simulink model "SistemaLineal"  (R2018b)
settings: Solver=VariableStepAuto  StartTime=0.0  StopTime=ttotal  RelTol=1e-3
values from neighbouring files (symbols this model uses):
  denom = conv(conv(conv([1 0.2], [1 -0.6]),[1 0.4]),[1 -0.1])    [PruebaMinCuadrados.m]
  num = conv(conv(conv([1 0.5], [1 0.7]),[1 -0.2]),[0 1])    [PruebaMinCuadrados.m]
  tmuestra = 0.05    [IDDATA.m]    (also in Identificacion.m; PruebaMinCuadrados.m)
  var = 0.00001    (= 1e-05)    [Identificacion.m]    (also in PruebaMinCuadrados.m = 0.001)
undefined symbols (not defined in the file or in its folder): iseed
settings Model: Creator=pablo  LastModifiedBy=pablo

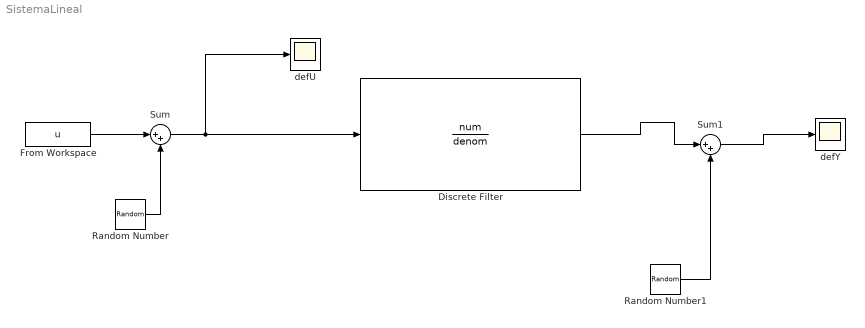
== system SistemaLineal ==
  Discrete Filter : DiscreteFilter  Numerator=num  Denominator=denom
  From Workspace : FromWorkspace  VariableName=u  SampleTime=tmuestra
  Random Number : RandomNumber  Variance=var  Seed=354872  SampleTime=tmuestra
  Random Number1 : RandomNumber  Variance=var/10000  Seed=iseed  SampleTime=tmuestra
  Sum : Sum  Inputs=|++
  Sum1 : Sum  Inputs=|++
  "defU " : Scope
  "defY " : Scope
  wires:
  From Workspace/1 -> Sum/1
  Random Number/1 -> Sum/2
  Sum/1 -> Discrete Filter/1, "defU "/1
  Random Number1/1 -> Sum1/2
  Discrete Filter/1 -> Sum1/1
  Sum1/1 -> "defY "/1
